simulink model "dovomi"  (R2016b)
settings: Solver=ode4  StartTime=0.0  StopTime=1200  FixedStep=0.01  RelTol=1e-3
settings Model: Creator=diamond  LastModifiedBy=diamond

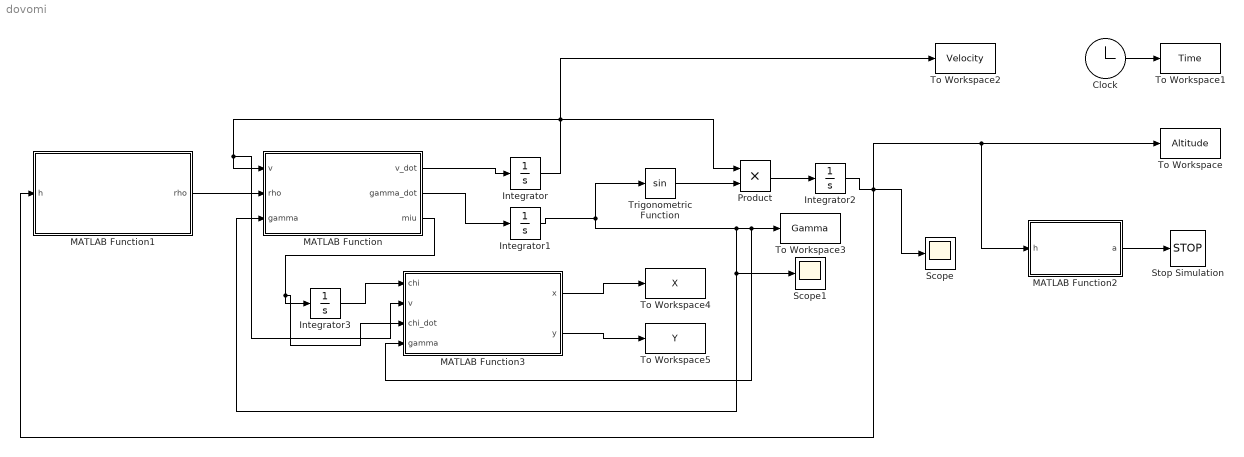
== system dovomi ==
  Clock : Clock
  Integrator : Integrator  InitialCondition=233
  Integrator1 : Integrator  InitialCondition=-0.05
  Integrator2 : Integrator  InitialCondition=13000
  Integrator3 : Integrator  InitialCondition=-0.06
  MATLAB Function : MATLAB Function  TreatAsAtomicUnit=on
  MATLAB Function1 : MATLAB Function  TreatAsAtomicUnit=on
  MATLAB Function2 : MATLAB Function  TreatAsAtomicUnit=on
  MATLAB Function3 : MATLAB Function  TreatAsAtomicUnit=on
  Product : Product
  Scope : Scope
  Scope1 : Scope
  Stop Simulation : Stop
  To Workspace : ToWorkspace  VariableName=Altitude  SampleTime=-1
  To Workspace1 : ToWorkspace  VariableName=Time  SampleTime=-1
  To Workspace2 : ToWorkspace  VariableName=Velocity  SampleTime=-1
  To Workspace3 : ToWorkspace  VariableName=Gamma  SampleTime=-1
  To Workspace4 : ToWorkspace  VariableName=X  SampleTime=-1
  To Workspace5 : ToWorkspace  VariableName=Y  SampleTime=-1
  Trigonometric Function : Trigonometry
  wires:
  MATLAB Function/1(v_dot) -> Integrator/1
  MATLAB Function/2(gamma_dot) -> Integrator1/1
  Integrator/1 -> To Workspace2/1, Product/1, MATLAB Function3/2(v), MATLAB Function/1(v)
  Integrator1/1 -> MATLAB Function/3(gamma), Scope1/1, MATLAB Function3/4(gamma), To Workspace3/1, Trigonometric Function/1
  Trigonometric Function/1 -> Product/2
  Product/1 -> Integrator2/1
  Integrator2/1 -> Scope/1, MATLAB Function1/1(h), MATLAB Function2/1(h), To Workspace/1
  MATLAB Function1/1(rho) -> MATLAB Function/2(rho)
  Clock/1 -> To Workspace1/1
  MATLAB Function2/1(a) -> Stop Simulation/1
  MATLAB Function/3(miu) -> MATLAB Function3/3(chi_dot), Integrator3/1
  MATLAB Function3/1(x) -> To Workspace4/1
  MATLAB Function3/2(y) -> To Workspace5/1
  Integrator3/1 -> MATLAB Function3/1(chi)

== matlab function dovomi/MATLAB Function1 ==
  data: h input; rho output
function rho=func2(h)
g=9.81;
rho_sl=1.2256;
Tsl=288.15;
R=287;
T11=216.65;
rho11=0.36;
L=-0.0065;

if h<=11000
    rho=rho_sl*((Tsl + L*h)/Tsl)^(4.256);
else
    rho=rho11*exp((-g/(R*T11))*(h-11000));
end
end

== matlab function dovomi/MATLAB Function ==
  data: v input; v_dot output; rho input; gamma input; gamma_dot output; miu output
function [v_dot,gamma_dot,miu]=func(v,rho,gamma)
M=73500;
g=9.81;
W=M*g;
s=122.4;
chi_dot=0.02;

alpha=4*(pi/180);
Cl0=0.24;
Cl_alpha=5.19;
Cd0=0.024;
k=0.041;
Cl=Cl0+Cl_alpha*alpha;
Cd=Cd0+k*Cl^2; 
q=0.5*rho*v^2;
L=q*s*Cl;
D=q*s*Cd;
v_dot=(-D-(W*sin(gamma)))/M;
miu=asin((chi_dot*M*v*cos(gamma))/(L));
gamma_dot=(L*cos(miu)-W*cos(gamma))/(M*v);
%chi_dot=(L*sin(gamma))/(M*v*cos(gamma));
end

== matlab function dovomi/MATLAB Function2 ==
  data: h input; a output
function a=func(h)
if h==0
    a=1;
else
    a=0;
end
end

== matlab function dovomi/MATLAB Function3 ==
  data: chi input; x output; v input; chi_dot input; y output; gamma input
function [x,y]=func2(chi,v,chi_dot,gamma)
R=(v*cos(gamma))/chi_dot;
x=R*cos(chi);
y=R*sin(chi);
end
